simulink model "HSGModel"  (R2025b)
settings: Solver=FixedStepAuto  StartTime=0.0  StopTime=1.5  FixedStep=1e-6  MaxStep=1e-3  MinStep=1e-8  RelTol=1e-4
undefined symbols (not defined in the file or in its folder): cb, cc, cg, cs, Er, kb, ke, ki, ks, kt, L, L_DC, ms, mu, R, Rv, vd
libraries: simulink x4
settings Model: SimulationMode=accelerator  Creator=khalid  LastModifiedBy=khalidwaleed
settings SolverCC: InitialStep=1e-5  ZeroCrossAlgorithm=Adaptive
settings DataIOCC: SaveTime=off
settings DebuggingCC: MaskedZcDiagnostic=none  IgnoredZcDiagnostic=none

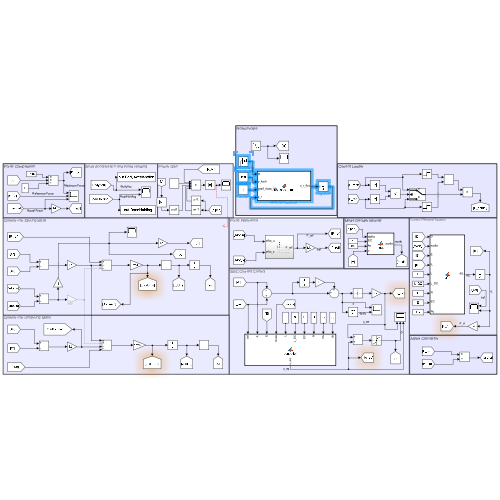
[thumbnail: Simulink's stored preview of the top-level diagram]
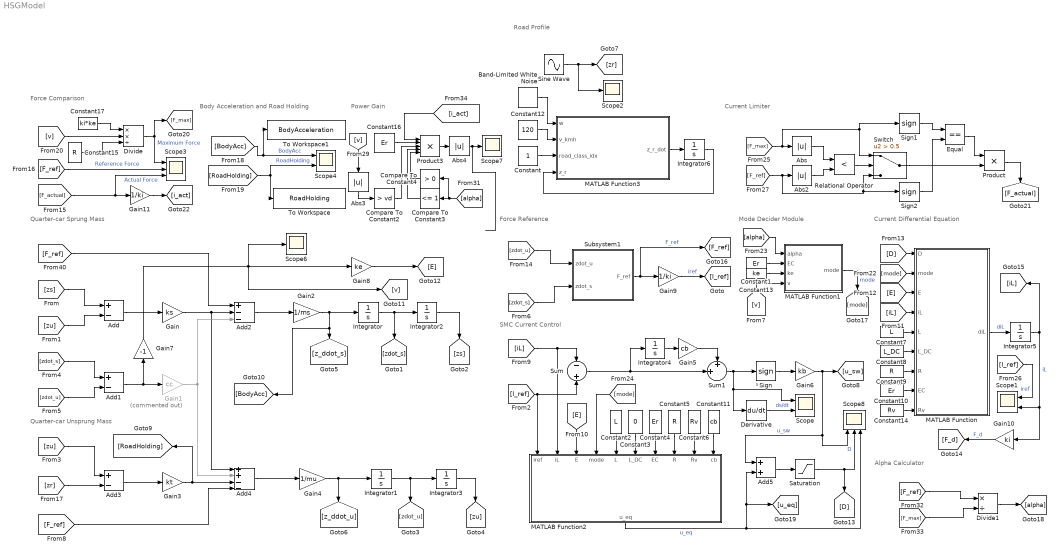
== system HSGModel ==
  note: Current Limiter
  note: Body Acceleration and Road Holding
  note: Force Comparison
  note: Alpha Calculator
  note: Mode Decider Module
  note: Current Differential Equation
  note: SMC Current Control
  note: Force Reference
  note: Quarter-car Sprung Mass
  note: Quarter-car Unsprung Mass
  note: Power Gain
  note: Road Profile
  Abs{,2..4} (4 alike) : Abs  SaturateOnIntegerOverflow=off
  Add : Sum  Inputs=+-
  Add1 : Sum  Inputs=+-
  Add2 : Sum  Inputs=+--
  Add3 : Sum  Inputs=+-
  Add4 : Sum  Inputs=++--
  Add5 : Sum
  Band-Limited White Noise : simulink/Sources/Band-Limited White Noise  Cov=[1]  Ts=0.01  seed=[23341]
  Compare To Constant2 : simulink/Logic and Bit Operations/Compare To Constant  relop=>  const=vd  OutDataTypeStr=uint8
  Compare To Constant3 : simulink/Logic and Bit Operations/Compare To Constant  relop=<=  const=1  OutDataTypeStr=uint8
  Compare To Constant4 : simulink/Logic and Bit Operations/Compare To Constant  relop=>  const=0  OutDataTypeStr=uint8
  Constant : Constant
  Constant{1,4,10,16} (4 alike) : Constant  Value=Er
  Constant11 : Constant  Value=cb
  Constant12 : Constant  Value=120
  Constant13 : Constant  Value=ke
  Constant14 : Constant  Value=Rv
  Constant15 : Constant  Value=R
  Constant17 : Constant  Value=ki*ke
  Constant2 : Constant  Value=L
  Constant3 : Constant  Value=0
  Constant5 : Constant  Value=R
  Constant6 : Constant  Value=Rv
  Constant7 : Constant  Value=L
  Constant8 : Constant  Value=L_DC
  Constant9 : Constant  Value=R
  Derivative : Derivative
  Divide : Product  Inputs=**/
  Divide1 : Product  Inputs=*/
  Equal : RelationalOperator  Operator===  OutDataTypeStr=boolean  RndMeth=Simplest  InputSameDT=off
  Gain : Gain  Gain=ks
  Gain1 : Gain  Commented=on  Gain=cc
  Gain10 : Gain  Gain=ki
  Gain11 : Gain  Gain=1/ki
  Gain2 : Gain  Gain=1/ms
  Gain3 : Gain  Gain=kt
  Gain4 : Gain  Gain=1/mu
  Gain5 : Gain  Gain=cb
  Gain6 : Gain  Gain=kb
  Gain7 : Gain  Gain=-1
  Gain8 : Gain  Gain=ke
  Gain9 : Gain  Gain=1/ki
  Integrator{,1..6} (7 alike) : Integrator
  MATLAB Function : MATLAB Function  TreatAsAtomicUnit=on
  MATLAB Function1 : MATLAB Function  TreatAsAtomicUnit=on
  MATLAB Function2 : MATLAB Function  TreatAsAtomicUnit=on
  MATLAB Function3 : MATLAB Function  TreatAsAtomicUnit=on
  Product : Product
  Product3 : Product  Inputs=5
  Relational Operator : RelationalOperator  Operator=<  OutDataTypeStr=boolean  RndMeth=Simplest  InputSameDT=off
  Saturation : Saturate  UpperLimit=1  LowerLimit=0
  Scope : Scope  NumInputPorts=2
      settings: ActiveDisplayYMinimum=-2.7447489042083522  ActiveDisplayYMaximum=2.8156790267575293  DataLoggingVariableName=ScopeData2
  Scope1 : Scope  NumInputPorts=2
      settings: ActiveDisplayYMinimum=-1  ActiveDisplayYMaximum=1
  Scope2 : Scope
      settings: ActiveDisplayYMinimum=-0.037499999999981493  ActiveDisplayYMaximum=0.037499999999892668
  Scope3 : Scope  NumInputPorts=3
      settings: ActiveDisplayYMinimum=-3070.1290805811605  ActiveDisplayYMaximum=3069.3182623125076  DataLoggingVariableName=ScopeData4
  Scope4 : Scope  NumInputPorts=2
      settings: ActiveDisplayYMinimum=-2.7443802906058909  ActiveDisplayYMaximum=2.7604562325107063  DataLoggingVariableName=ScopeData5
  Scope6 : Scope
      settings: ActiveDisplayYMinimum=-0.36866118759995997  ActiveDisplayYMaximum=0.40056532030192649  DataLoggingVariableName=ScopeData6
  Scope7 : Scope
      settings: ActiveDisplayYMinimum=-11.009223175045067  ActiveDisplayYMaximum=99.083008575405614  DataLoggingVariableName=ScopeData7
  Scope8 : Scope  NumInputPorts=3
      settings: ActiveDisplayYMinimum=-1.7651094697775311  ActiveDisplayYMaximum=2.8491770678518753  DataLoggingVariableName=ScopeData8
  Sign : Signum
  Sign1 : Signum
  Sign2 : Signum
  Sine Wave : Sin  Amplitude=0.03  Frequency=2*pi*1.3  SampleTime=0
  Subsystem1 : Subsystem
  Sum : Sum  Inputs=-+
  Sum1 : Sum  Inputs=+|+||
  Switch : Switch  Criteria=u2 > Threshold  Threshold=0.5  SaturateOnIntegerOverflow=off  InputSameDT=off
  To Workspace : ToWorkspace  VariableName=RoadHolding  SaveFormat=Structure With Time  SampleTime=-1
  To Workspace1 : ToWorkspace  VariableName=BodyAcceleration  SaveFormat=Structure With Time  SampleTime=-1
  wires:
  [zdot_u] -> Add1/2
  Add3/1 -> Gain3/1
  Gain3/1 -> [RoadHolding], Add4/3
  [zs] -> Add/1
  Add1/1 -> Gain1/1, Gain7/1
  [zr] -> Add3/2
  Add4/1 -> Gain4/1
  Integrator/1 -> Integrator2/1, [zdot_s]
  [zu] -> Add/2
  [F_ref] -> Add4/4
  [zdot_s] -> Add1/1
  Gain2/1 -> Integrator/1, [BodyAcc], [z_ddot_s]
  Gain/1 -> Add4/1, Add2/2
  Add/1 -> Gain/1
  Gain4/1 -> Integrator1/1, [z_ddot_u]
  [zu] -> Add3/1
  Add2/1 -> Gain2/1
  Integrator3/1 -> [zu]
  Integrator1/1 -> Integrator3/1, [zdot_u]
  Integrator2/1 -> [zs]
  [F_ref] -> Add2/1
  [BodyAcc] -> To Workspace1/1, Scope4/1  "BodyAcc"
  [RoadHolding] -> To Workspace/1, Scope4/2  "RoadHolding"
  [F_actual] -> Gain11/1, Scope3/3  "Actual Force"
  Divide/1 -> [F_max], Scope3/1  "Maximum Force"
  [F_ref] -> Scope3/2  "Reference Force"
  Constant15/1 -> Divide/3
  [zdot_u] -> Subsystem1/1(zdot_u)
  Subsystem1/1(F_ref) -> [F_ref], Gain9/1  "F_ref"
  [zdot_s] -> Subsystem1/2(zdot_s)
  Gain9/1 -> [I_ref]  "iref"
  [iL] -> MATLAB Function2/2(iL), Sum/1
  Sign/1 -> Gain6/1
  Integrator4/1 -> Gain5/1
  [I_ref] -> MATLAB Function2/1(iref), Sum/2
  Sum1/1 -> Derivative/1, Scope/1, Sign/1  "s"
  Gain6/1 -> Add5/1, Scope8/1, [u_sw]  "u_sw"
  Constant5/1 -> MATLAB Function2/8(R)
  Constant11/1 -> MATLAB Function2/10(cb)
  Constant3/1 -> MATLAB Function2/6(L_DC)
  Constant4/1 -> MATLAB Function2/7(EC)
  Constant6/1 -> MATLAB Function2/9(Rv)
  Constant2/1 -> MATLAB Function2/5(L)
  Gain8/1 -> [E]
  [E] -> MATLAB Function2/3(E)
  Add5/1 -> Saturation/1
  Saturation/1 -> Scope8/2, [D]  "D"
  Constant8/1 -> MATLAB Function/6(L_DC)
  Constant9/1 -> MATLAB Function/7(R)
  Integrator5/1 -> Scope1/2, Gain10/1, [iL]  "iL"
  MATLAB Function/1(diL) -> Integrator5/1  "diL"
  Gain10/1 -> [F_d]  "F_d"
  Constant14/1 -> MATLAB Function/9(Rv)
  Constant10/1 -> MATLAB Function/8(EC)
  Constant7/1 -> MATLAB Function/5(L)
  [iL] -> MATLAB Function/4(iL)
  [E] -> MATLAB Function/3(E)
  [D] -> MATLAB Function/1(D)
  Constant13/1 -> MATLAB Function1/3(ke)
  Constant1/1 -> MATLAB Function1/2(EC)
  [v] -> MATLAB Function1/4(v)
  MATLAB Function1/1(mode) -> [mode]  "mode"
  [mode] -> MATLAB Function/2(mode)
  [alpha] -> MATLAB Function1/1(alpha)
  [mode] -> MATLAB Function2/4(mode)
  Gain5/1 -> Sum1/1
  Constant17/1 -> Divide/1
  [v] -> Divide/2
  Abs/1 -> Relational Operator/1
  [F_ref] -> Sign2/1, Switch/3, Abs2/1
  Abs2/1 -> Relational Operator/2
  Relational Operator/1 -> Switch/2
  [F_max] -> Switch/1, Sign1/1, Abs/1
  [F_ref] -> Divide1/1
  [F_max] -> Divide1/2
  Divide1/1 -> [alpha]
  Gain7/1 -> Scope6/1, Gain8/1, [v]
  Derivative/1 -> Scope/2  "ds/dt"
  [I_ref] -> Scope1/1  "iref"
  Sign1/1 -> Equal/1
  Sign2/1 -> Equal/2
  Equal/1 -> Product/1
  Switch/1 -> Product/2
  Product/1 -> [F_actual]
  Sum/1 -> Integrator4/1, Sum1/2
  Gain11/1 -> [i_act]
  Gain1/1 -> Add4/2, Add2/3
  MATLAB Function2/1(u_eq) -> Add5/2, [u_eq], Scope8/3  "u_eq"
  Compare To Constant3/1 -> Product3/4
  Abs3/1 -> Compare To Constant2/1
  Compare To Constant2/1 -> Product3/3
  [v] -> Abs3/1
  [i_act] -> Product3/1
  [alpha] -> Compare To Constant4/1, Compare To Constant3/1
  Compare To Constant4/1 -> Product3/5
  Band-Limited White Noise/1 -> MATLAB Function3/1(w)
  MATLAB Function3/1(z_r_dot) -> Integrator6/1
  Constant12/1 -> MATLAB Function3/2(v_kmh)
  Constant/1 -> MATLAB Function3/3(road_class_idx)
  Integrator6/1 -> MATLAB Function3/4(z_r)
  Constant16/1 -> Product3/2
  Abs4/1 -> Scope7/1
  Product3/1 -> Abs4/1
  Sine Wave/1 -> Scope2/1, [zr]

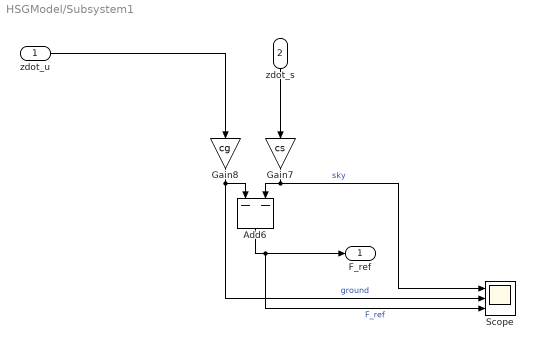
== system HSGModel/Subsystem1 ==
  zdot_u : Inport
  zdot_s : Inport  Port=2
  Add6 : Sum  Inputs=--
  Gain7 : Gain  Gain=cs
  Gain8 : Gain  Gain=cg
  Scope : Scope  NumInputPorts=3
      settings: ActiveDisplayYMinimum=-234.54288401118075  ActiveDisplayYMaximum=232.10620472540066  DataLoggingVariableName=ScopeData10
  F_ref : Outport
  wires:
  Gain8/1 -> Scope/2, Add6/1  "ground"
  Gain7/1 -> Add6/2, Scope/1  "sky"
  zdot_s/1 -> Gain7/1
  Add6/1 -> Scope/3, F_ref/1  "F_ref"
  zdot_u/1 -> Gain8/1

== matlab function HSGModel/MATLAB Function1 ==
  data: alpha input; EC input; ke input; v input; mode output
function mode = mode(alpha, EC, ke, v)

    % guard against alpha >= 1
    if alpha >= 1
        % semi-active not achievable
        % both VT1 and VT2 on, passive damper
        mode = 1;   % or handle separately
        return
    end

    v_alpha = EC / (ke * (1 - alpha));

    if abs(v) < v_alpha
        mode = 1;   % boost
    else
        mode = 0;   % buck
    end
end

== matlab function HSGModel/MATLAB Function ==
  data: D input; mode input; E input; iL input; diL output; L input; L_DC input; R input; EC input; Rv input
function diL = diL(D, mode, E, iL, L, L_DC, R, EC, Rv)
    LDC = L + L_DC;
    if mode == 1  % boost
        diL = -(R/LDC)*iL - ((1-D)/LDC)*EC + (1/LDC)*E;
    else          % buck
        diL  = -((D*R*L + (1-D)*(R+Rv)*LDC)/(L * LDC))*iL - (D/LDC)*EC + (D*L + (1-D)*LDC)/(L * LDC) * E;
    end
end

== matlab function HSGModel/MATLAB Function2 ==
  data: iref input; iL input; E input; mode input; u_eq output; L input; L_DC input; EC input; R input; Rv input; cb input
function u_eq = controller(iref, iL, E, mode, L, L_DC, EC, R, Rv, cb)
    LDC = L + L_DC;
    e   = iref - iL;        % current error

    if mode == 1  % boost
        numerator   = EC - E + R*iref + cb*e*LDC;
        denominator = EC;
        u_eq = numerator / denominator;

    else          % buck
        numerator   = E - (R + Rv)*iref - cb*e*L;
        denominator = (L*R*iref)/LDC - (R + Rv)*iref + ((EC - E)*L)/LDC + E;
        u_eq = numerator / denominator;
    end
end

== matlab function HSGModel/MATLAB Function3 ==
  data: w input; z_r_dot output; v_kmh input; road_class_idx input; z_r input
function z_r_dot = iso_road_filter(w, v_kmh, road_class_idx, z_r)
    % Inputs:
    %   w              - White noise input signal
    %   v_kmh          - Vehicle speed in km/h from workspace
    %   road_class_idx - 1 for Class B, 2 for Class D
    %   z_r            - Current road displacement (feedback loop)
    
    % Constants
    n_0 = 0.1;   % Reference spatial frequency (cycles/m)
    n_c = 0.01;  % Low frequency cut-off (cycles/m)
    
    % Convert speed from km/h to m/s
    v = v_kmh / 3.6; 
    
    % Select roughness coefficient based on road class index
    if road_class_idx == 1
        G_0 = 64e-6;   % Class B nominal
    else
        G_0 = 1024e-6; % Class D nominal
    end
    
    % Avoid division by zero if vehicle stops
    if v < 0.1
        v = 0.1;
    end
    
    % Compute the derivative of the road profile displacement
    z_r_dot = -2*pi*n_c*v*z_r + 2*pi*n_0*sqrt(G_0*v)*w;
end
